simulink model "Sub_System"  (R2020b)
settings: Solver=VariableStepAuto  StartTime=0.0  StopTime=10.0  RelTol=1e-3
undefined symbols (not defined in the file): b, ki, kp, m
settings Model: Creator=vikas  LastModifiedBy=sonal

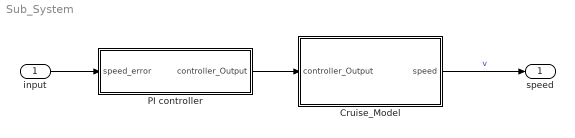
== system Sub_System ==
  input : Inport  OutDataTypeStr=double  PortDimensions=1  SampleTime=0
  Cruise_Model : Subsystem
  PI controller : Subsystem
  speed : Outport  OutDataTypeStr=double  PortDimensions=1  SampleTime=0
  wires:
  PI controller/1(controller_Output) -> Cruise_Model/1(controller_Output)
  Cruise_Model/1(speed) -> speed/1  "v"
  input/1 -> PI controller/1(speed_error)

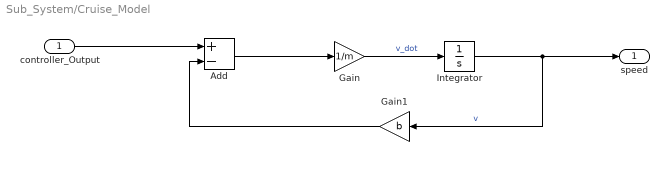
== system Sub_System/Cruise_Model ==
  controller_Output : Inport
  Add : Sum  Inputs=+-
  Gain : Gain  Gain=1/m
  Gain1 : Gain  Gain=b
  Integrator : Integrator
  speed : Outport
  wires:
  controller_Output/1 -> Add/1
  Integrator/1 -> Gain1/1, speed/1  "v"
  Gain/1 -> Integrator/1  "v_dot"
  Gain1/1 -> Add/2
  Add/1 -> Gain/1

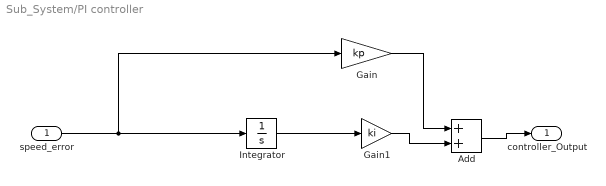
== system Sub_System/PI controller ==
  speed_error : Inport
  Add : Sum
  Gain : Gain  Gain=kp
  Gain1 : Gain  Gain=ki
  Integrator : Integrator
  controller_Output : Outport
  wires:
  speed_error/1 -> Integrator/1, Gain/1
  Integrator/1 -> Gain1/1
  Gain/1 -> Add/1
  Add/1 -> controller_Output/1
  Gain1/1 -> Add/2
